simulink model "ATRIAS_vnmc"  (R2015a)
settings: Solver=ode45  StartTime=0.0  StopTime=60  FixedStep=1e-3  MinStep=1e-6  RelTol=1e-3  AbsTol=1e-4
values from neighbouring files (symbols this model uses):
  initial_boom_yaw = initial_boom_yaw + delta_yaw0    [run_model.m]
  max_floor_diff = cost_fun_opts.max_floor_diff    [opt_cmaes.m]    (also in run_model.m; set_all_params_simple.m = 0)
  noise_on_off = cost_fun_opts.noise_on_off    [opt_cmaes.m]    (also in run_model.m; set_all_params_simple.m = 0)
  noise_seed = cost_fun_opts.noise_seed    [opt_cmaes.m]    (also in run_model.m; set_all_params_simple.m = 1)
  noise_variance = cost_fun_opts.noise_variance    [opt_cmaes.m]    (also in run_model.m; set_all_params_simple.m = 0.000174532925199)
  SEA_swing_ctrl_on_off = cost_fun_opts.SEA_swing_ctrl_on_off    [opt_cmaes.m]    (also in run_model.m; set_all_params_simple.m = 0)
  sim_t = simout.twalk    [run_model.m]
  steady_dist = cost_fun_opts.steady_dist    [opt_cmaes.m]    (also in run_model.m; set_all_params_simple.m = 10)
  ts_anim = 0.0333    [run_model.m]
undefined symbols (not defined in the file or in its folder): A1_notch_f1, A2_notch_f1, A_lpf_dtau, A_lpf_velocity, B1_lpf_dtau, B1_lpf_velocity, B1_notch_f1, B2_lpf_dtau, B2_lpf_velocity, B2_notch_f1, b_hmotor, b_leg_spring, b_rotor, base_color_d, boom_color_d, boom_mount_to_center_diagonal, breakaway_friction, c, c_jointstop, com_height_offset, contactThr, coulomb_friction, CtrlPar_theta0, D12_S, D12_T, d_com, ddx_max, ddy_max, delta_phi_max, delta_phi_max_buffer, delta_phi_max_dropoff, delta_phi_min, des_forward_velocity, DS_width, dtau_des_max, dtheta0_vmc, dx0_vmc, dy_max, eref, fblink_color_d, fcut_acceleration, floor_color_d, floor_tile_width, floor_zero_height, FmaxBFSH, FmaxGLU, FmaxHAM, FmaxHFL, FmaxRF, FmaxVAS, FPCtrlPar, friction_linear_zone, g, gain_nodes_sea_torque, gamma_stance_thr, gamma_swing_thr, hip_height, HIP_MTR_MAX_CONT_TORQUE, HIP_MTR_MAX_TORQUE, hshaft_color_d ... (+236)
libraries: sm_lib x280, nesl_utility x174, simulink x114, simulink_extras x58, fl_lib x16, mblibv1 x2, dspswit3 x2
(part 2 of 23)

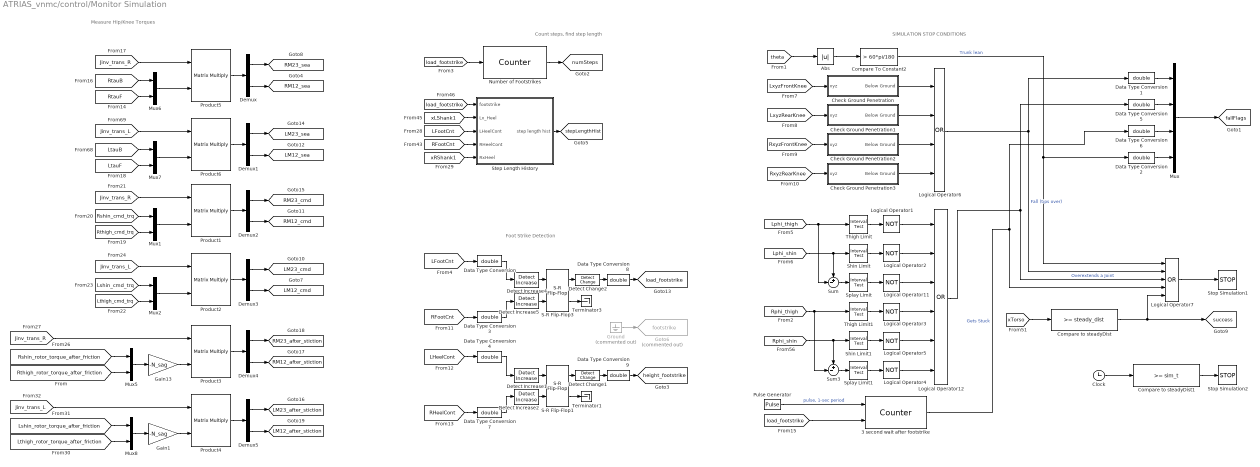
== system ATRIAS_vnmc/control/Monitor Simulation ==
  note: Foot Strike Detection
  note: Count steps, find step length
  note: SIMULATION STOP CONDITIONS
  note: Measure Hip/Knee Torques
  3 second wait after footstrike : dspswit3/Counter  Direction=Up  CountEvent=Rising edge  CounterSize=User defined  MaxCount=255  InitialCount=0  Output=Hit  HitValue=4  ResetInput=on  SamplesPerFrame=1  Ts=1  CntDtype=double  HitDtype=Boolean
  Abs : Abs
  Check Ground Penetration : Subsystem
  Check Ground Penetration1 : Subsystem
  Check Ground Penetration2 : Subsystem
  Check Ground Penetration3 : Subsystem
  Clock : Clock
  Compare To Constant2 : simulink/Logic and Bit Operations/Compare To Constant  relop=>  const=60*pi/180  OutDataTypeStr=boolean
  Compare to steadyDist : simulink/Logic and Bit Operations/Compare To Constant  relop=>=  const=steady_dist  OutDataTypeStr=boolean
  Compare to steadyDist1 : simulink/Logic and Bit Operations/Compare To Constant  relop=>=  const=sim_t  OutDataTypeStr=boolean
  Data Type Conversion{,1..9} (10 alike) : DataTypeConversion  OutDataTypeStr=double
  Demux{,1..5} (6 alike) : Demux  Outputs=2
  Detect Change1 : simulink/Logic and Bit Operations/Detect Change  vinit=0  InputProcessing=Inherited  OutDataTypeStr=boolean
  Detect Change2 : simulink/Logic and Bit Operations/Detect Change  vinit=0  InputProcessing=Inherited  OutDataTypeStr=boolean
  Detect Increase{1..2,4..5} (4 alike) : simulink/Logic and Bit Operations/Detect Increase  vinit=0.0  InputProcessing=Inherited  OutDataTypeStr=boolean
  Gain1 : Gain  Gain=-N_sag
  Gain13 : Gain  Gain=-N_sag
  Goto6 : Goto  Commented=on  GotoTag=footstrike  TagVisibility=global
  Ground : Ground  Commented=on
  Logical Operator{1..5,11} (6 alike) : Logic  Operator=NOT  AllPortsSameDT=off  OutDataTypeStr=boolean
  Logical Operator12 : Logic  Operator=OR  Inputs=6  AllPortsSameDT=off  OutDataTypeStr=boolean
  Logical Operator6 : Logic  Operator=OR  Inputs=4  AllPortsSameDT=off  OutDataTypeStr=boolean
  Logical Operator7 : Logic  Operator=OR  Inputs=5  AllPortsSameDT=off  OutDataTypeStr=boolean
  Mux : Mux
  Mux{1..2,5..8} (6 alike) : Mux  Inputs=2
  Number of Footstrikes : dspswit3/Counter  Direction=Up  CountEvent=Rising edge  CounterSize=User defined  MaxCount=255  InitialCount=0  Output=Count  HitValue=4  ResetInput=off  SamplesPerFrame=1  Ts=1  CntDtype=double  HitDtype=Boolean
  Product{1..6} (6 alike) : Product  Multiplication=Matrix(*)  InputSameDT=on
  Pulse Generator : DiscretePulseGenerator  PulseType=Time based  Period=1  PulseWidth=5
  S-R Flip-Flop1 : simulink_extras/Flip Flops/S-R Flip-Flop  initial_condition=1
  S-R Flip-Flop3 : simulink_extras/Flip Flops/S-R Flip-Flop  initial_condition=1
  Shin Limit : simulink/Logic and Bit Operations/Interval Test  IntervalClosedRight=on  uplimit=phi_shin_max  IntervalClosedLeft=on  lowlimit=phi_shin_min  OutDataTypeStr=boolean
  Shin Limit1 : simulink/Logic and Bit Operations/Interval Test  IntervalClosedRight=on  uplimit=phi_shin_max  IntervalClosedLeft=on  lowlimit=phi_shin_min  OutDataTypeStr=boolean
  Splay Limit : simulink/Logic and Bit Operations/Interval Test  IntervalClosedRight=on  uplimit=delta_phi_max  IntervalClosedLeft=on  lowlimit=delta_phi_min  OutDataTypeStr=boolean
  Splay Limit1 : simulink/Logic and Bit Operations/Interval Test  IntervalClosedRight=on  uplimit=delta_phi_max  IntervalClosedLeft=on  lowlimit=delta_phi_min  OutDataTypeStr=boolean
  Step Length History : Subsystem
  Stop Simulation1 : Stop
  Stop Simulation2 : Stop
  Sum : Sum  Inputs=+-|
  Sum3 : Sum  Inputs=+-|
  Terminator1 : Terminator
  Terminator3 : Terminator
  Thigh Limit : simulink/Logic and Bit Operations/Interval Test  IntervalClosedRight=on  uplimit=phi_thigh_max  IntervalClosedLeft=on  lowlimit=phi_thigh_min  OutDataTypeStr=boolean
  Thigh Limit1 : simulink/Logic and Bit Operations/Interval Test  IntervalClosedRight=on  uplimit=phi_thigh_max  IntervalClosedLeft=on  lowlimit=phi_thigh_min  OutDataTypeStr=boolean
  tag scope: LM12_after_stiction=global, LM12_cmd=global, LM12_sea=global, LM23_after_stiction=global, LM23_cmd=global, LM23_sea=global, RM12_after_stiction=global, RM12_cmd=global, RM12_sea=global, RM23_after_stiction=global, RM23_cmd=global, RM23_sea=global, fallFlags=global, height_footstrike=global, load_footstrike=global, numSteps=global, stepLengthHist=global, success=global
  wires:
  [theta] -> Abs/1
  Mux/1 -> [fallFlags]
  Pulse Generator/1 -> 3 second wait after footstrike/1  "pulse, 1-sec period"
  [load_footstrike] -> 3 second wait after footstrike/2
  Logical Operator6/1 -> Logical Operator7/2, Data Type Conversion1/1  "Fall (tips over)"
  Logical Operator12/1 -> Logical Operator7/3, Data Type Conversion5/1  "Overextends a Joint"
  3 second wait after footstrike/1 -> Logical Operator7/4, Data Type Conversion6/1  "Gets Stuck"
  [load_footstrike] -> Number of Footstrikes/1
  Number of Footstrikes/1 -> [numSteps]
  [load_footstrike] -> Step Length History/1(footstrike)
  [xLShank1] -> Step Length History/2(Lx_Heel)
  [LFootCnt] -> Step Length History/3(LHeelCont)
  [RFootCnt] -> Step Length History/4(RHeelCont)
  [xRShank1] -> Step Length History/5(RxHeel)
  Step Length History/1(step length hist) -> [stepLengthHist]
  [xTorso] -> Compare to steadyDist/1
  Compare to steadyDist/1 -> Logical Operator7/5, [success]
  Logical Operator7/1 -> Stop Simulation1/1
  Splay Limit/1 -> Logical Operator11/1
  Thigh Limit/1 -> Logical Operator1/1
  Shin Limit/1 -> Logical Operator2/1
  Logical Operator1/1 -> Logical Operator12/1
  Logical Operator2/1 -> Logical Operator12/2
  Logical Operator11/1 -> Logical Operator12/3
  Logical Operator3/1 -> Logical Operator12/4
  Logical Operator5/1 -> Logical Operator12/5
  Logical Operator4/1 -> Logical Operator12/6
  Splay Limit1/1 -> Logical Operator4/1
  Thigh Limit1/1 -> Logical Operator3/1
  Shin Limit1/1 -> Logical Operator5/1
  [Lphi_thigh] -> Thigh Limit/1, Sum/2
  [Lphi_shin] -> Shin Limit/1, Sum/1
  Sum/1 -> Splay Limit/1
  [Rphi_thigh] -> Sum3/2, Thigh Limit1/1
  [Rphi_shin] -> Sum3/1, Shin Limit1/1
  Sum3/1 -> Splay Limit1/1
  [LxyzFrontKnee] -> Check Ground Penetration/1(xyz)
  [RxyzRearKnee] -> Check Ground Penetration3/1(xyz)
  [RxyzFrontKnee] -> Check Ground Penetration2/1(xyz)
  [LxyzRearKnee] -> Check Ground Penetration1/1(xyz)
  Check Ground Penetration/1(Below Ground) -> Logical Operator6/1
  Check Ground Penetration1/1(Below Ground) -> Logical Operator6/2
  Check Ground Penetration2/1(Below Ground) -> Logical Operator6/3
  Check Ground Penetration3/1(Below Ground) -> Logical Operator6/4
  Compare To Constant2/1 -> Logical Operator7/1, Data Type Conversion2/1  "Trunk lean"
  Data Type Conversion1/1 -> Mux/1
  Data Type Conversion6/1 -> Mux/3
  Data Type Conversion5/1 -> Mux/2
  Data Type Conversion2/1 -> Mux/4
  Abs/1 -> Compare To Constant2/1
  [LFootCnt] -> Data Type Conversion/1
  [RFootCnt] -> Data Type Conversion3/1
  Detect Increase4/1 -> S-R Flip-Flop3/1
  Detect Increase5/1 -> S-R Flip-Flop3/2
  Detect Change2/1 -> Data Type Conversion8/1
  S-R Flip-Flop3/1 -> Detect Change2/1
  S-R Flip-Flop3/2 -> Terminator3/1
  Data Type Conversion8/1 -> [load_footstrike]
  Data Type Conversion/1 -> Detect Increase4/1
  Data Type Conversion3/1 -> Detect Increase5/1
  [LHeelCont] -> Data Type Conversion4/1
  [RHeelCont] -> Data Type Conversion7/1
  Detect Increase1/1 -> S-R Flip-Flop1/1
  Detect Increase2/1 -> S-R Flip-Flop1/2
  Detect Change1/1 -> Data Type Conversion9/1
  S-R Flip-Flop1/1 -> Detect Change1/1
  S-R Flip-Flop1/2 -> Terminator1/1
  Data Type Conversion9/1 -> [height_footstrike]
  Data Type Conversion4/1 -> Detect Increase1/1
  Data Type Conversion7/1 -> Detect Increase2/1
  Ground/1 -> Goto6/1
  [RtauB] -> Mux6/1
  [RtauF] -> Mux6/2
  Mux6/1 -> Product5/2
  [Jinv_trans_R] -> Product5/1
  Product5/1 -> Demux/1
  Demux/2 -> [RM12_sea]
  Demux/1 -> [RM23_sea]
  [LtauB] -> Mux7/1
  [LtauF] -> Mux7/2
  Mux7/1 -> Product6/2
  [Jinv_trans_L] -> Product6/1
  Product6/1 -> Demux1/1
  Demux1/2 -> [LM12_sea]
  Demux1/1 -> [LM23_sea]
  [Rshin_cmd_trq] -> Mux1/1
  [Rthigh_cmd_trq] -> Mux1/2
  Mux1/1 -> Product1/2
  [Jinv_trans_R] -> Product1/1
  Product1/1 -> Demux2/1
  Demux2/2 -> [RM12_cmd]
  Demux2/1 -> [RM23_cmd]
  [Lshin_cmd_trq] -> Mux2/1
  [Lthigh_cmd_trq] -> Mux2/2
  Mux2/1 -> Product2/2
  [Jinv_trans_L] -> Product2/1
  Product2/1 -> Demux3/1
  Demux3/2 -> [LM12_cmd]
  Demux3/1 -> [LM23_cmd]
  Clock/1 -> Compare to steadyDist1/1
  Compare to steadyDist1/1 -> Stop Simulation2/1
  [Jinv_trans_R] -> Product3/1
  Product3/1 -> Demux4/1
  Demux4/2 -> [RM12_after_stiction]
  Demux4/1 -> [RM23_after_stiction]
  [Jinv_trans_L] -> Product4/1
  Product4/1 -> Demux5/1
  Demux5/2 -> [LM12_after_stiction]
  Demux5/1 -> [LM23_after_stiction]
  [Rshin_rotor_torque_after_friction] -> Mux5/1
  [Rthigh_rotor_torque_after_friction] -> Mux5/2
  Mux5/1 -> Gain13/1
  [Lshin_rotor_torque_after_friction] -> Mux8/1
  [Lthigh_rotor_torque_after_friction] -> Mux8/2
  Mux8/1 -> Gain1/1
  Gain13/1 -> Product3/2
  Gain1/1 -> Product4/2

== system ATRIAS_vnmc/control/Plot Signals ==
  note: Virtual Torques
  note: GRFs, Leg Load,
      | Contact
  note: Virtual Joint Angles
  note: Robot Joint Angles
  note: Joint Torques
  note: Global Marker Positions
  note: Muscle States
  note: Individual Muscles
  note: Stimulations
  note: Muscle Lce,
      | Moment Arms
  note: Compare Continuous
      | to Discrete Angles
  note: VMC
  Discrete-Continuous Plots : Subsystem
  "GRFs, leg load, contact" : Subsystem
  Markers : Subsystem
  Robot Angles : Subsystem
  Torques : Subsystem
  VMC Plots : Subsystem
  Virtual Angles : Subsystem
  individual muscles : Subsystem
  muscle comparison : Subsystem
  muscle etc : Subsystem
  stims : Subsystem  Commented=on
  virtual joint torques : Subsystem

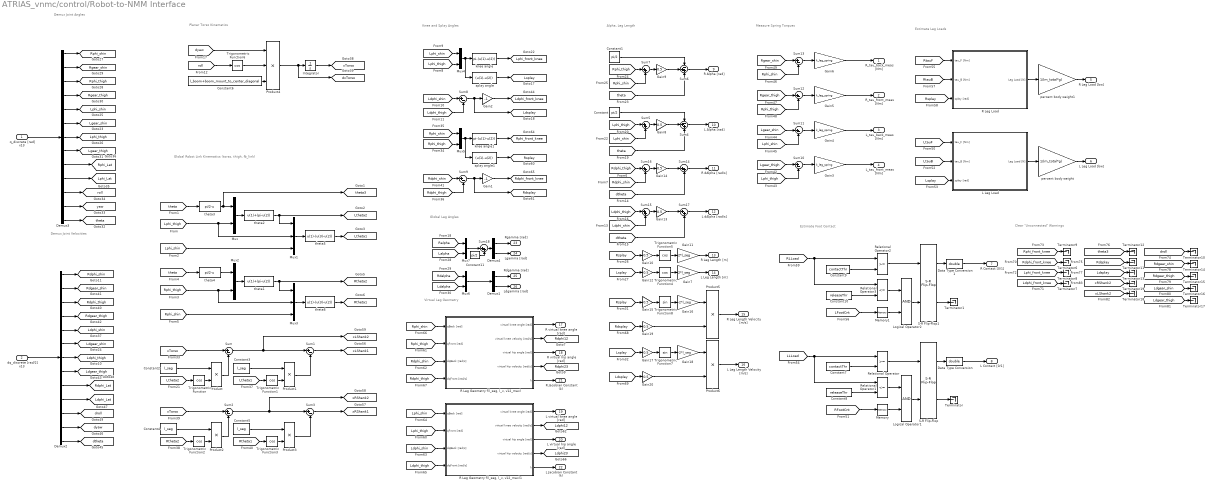
== system ATRIAS_vnmc/control/Robot-to-NMM Interface ==
  note: Global Robot Link Kinematics
      | (torso, thigh, fb_link)
  note: Planar Torso Kinematics
  note: Alpha, Leg Length
  note: Demux Joint
      | Angles
  note: Demux Joint
      | Velocities
  note: Knee and Splay Angles
  note: Virtual Leg Geometry
  note: Measure Spring Torques
  note: Estimate Leg Loads
  note: Estimate Foot Contact
  note: Clear "Unconnected" Warnings
  note: Global Leg Angles
  q_discrete [rad] x13 : Inport
  dq_discrete [rad/2] x13 : Inport  Port=2
  Constant : Constant  Value=pi/2
  Constant1 : Constant  Value=pi/2
  Constant10 : Constant  Value=releaseThr
  Constant11 : Constant  Value=pi/2
  Constant{2..5} (4 alike) : Constant  Value=l_seg
  Constant6 : Constant  Value=l_boom+boom_mount_to_center_diagonal
  Constant7 : Constant  Value=contactThr
  Constant8 : Constant  Value=releaseThr
  Constant9 : Constant  Value=contactThr
  Data Type Conversion : DataTypeConversion  OutDataTypeStr=double
  Data Type Conversion1 : DataTypeConversion  OutDataTypeStr=double
  Demux1 : Demux  Outputs=2
  Demux2 : Demux  Outputs=13
  Demux3 : Demux  Outputs=13
  Demux4 : Demux  Outputs=2
  Gain1 : Gain  Gain=-1
  Gain{8..10,12..15,17,19..20} (10 alike) : Gain  Gain=0.5
  Gain11 : Gain  Gain=2*l_seg
  Gain16 : Gain  Gain=-2*l_seg
  Gain18 : Gain  Gain=-2*l_seg
  Gain2 : Gain  Gain=-1
  Gain{3..6} (4 alike) : Gain  Gain=k_leg_spring
  Gain7 : Gain  Gain=2*l_seg
  Integrator : Integrator
  L Leg Load : Subsystem
  Logical Operator1 : Logic  AllPortsSameDT=off  OutDataTypeStr=boolean
  Logical Operator2 : Logic  AllPortsSameDT=off  OutDataTypeStr=boolean
  Memory : Memory
  Memory1 : Memory
  Mux{,2,4..7} (6 alike) : Mux  Inputs=2
  Mux1 : Mux  Inputs=3
  Mux3 : Mux  Inputs=3
  Product{,1..3,5..6} (6 alike) : Product
  Product4 : Product  Inputs=3
  "R Leg Geometry f(l_seg, l_v, v12_max)" : Subsystem
  "R Leg Geometry f(l_seg, l_v, v12_max)1" : Subsystem
  R Leg Load : Subsystem
  Relational Operator : RelationalOperator  OutDataTypeStr=boolean
  Relational Operator1 : RelationalOperator  Operator=<=  OutDataTypeStr=boolean
  Relational Operator2 : RelationalOperator  OutDataTypeStr=boolean
  Relational Operator3 : RelationalOperator  Operator=<=  OutDataTypeStr=boolean
  S-R Flip-Flop : simulink_extras/Flip Flops/S-R Flip-Flop  initial_condition=0
  S-R Flip-Flop1 : simulink_extras/Flip Flops/S-R Flip-Flop  initial_condition=0
  Sum{,1..3,8..13} (10 alike) : Sum  Inputs=|+-
  Sum{5,7,14..18} (7 alike) : Sum  Inputs=|++
  Sum4 : Sum  Inputs=-++
  Sum6 : Sum  Inputs=-++
  Terminator{,1,6..19} (16 alike) : Terminator
  Trigonometric Function{,1..6} (7 alike) : Trigonometry  Operator=cos
  Trigonometric Function7 : Trigonometry
  Trigonometric Function8 : Trigonometry
  knee angle : Fcn  Expr=pi-(u(1)-u(2))
  knee angle1 : Fcn  Expr=pi-(u(1)-u(2))
  percent body weight : Gain  Gain=1/(m_total*g)
  percent body weight1 : Gain  Gain=1/(m_total*g)
  splay angle : Fcn  Expr=(u(1)-u(2))
  splay angle1 : Fcn  Expr=(u(1)-u(2))
  theta1 : Fcn  Expr=u(1)+(pi-u(2))
  theta2 : Fcn  Expr=u(1)+(pi-u(2))
  theta3 : Fcn  Expr=pi/2-u
  theta4 : Fcn  Expr=pi/2-u
  theta5 : Fcn  Expr=u(1)-(u(3)-u(2))
  theta6 : Fcn  Expr=u(1)-(u(3)-u(2))
  R_tau_back_meas [Nm] : Outport
  R_tau_front_meas [Nm] : Outport  Port=2
  L_tau_back_meas [Nm] : Outport  Port=3
  L_tau_front_meas [Nm] : Outport  Port=4
  R Leg Load [bw] : Outport  Port=5
  L Leg Load [bw] : Outport  Port=6
  R Contact [0/1] : Outport  Port=7
  L Contact [0/1] : Outport  Port=8
  R Alpha [rad] : Outport  Port=9
  L Alpha [rad] : Outport  Port=10
  R dAlpha [rad/s] : Outport  Port=11
  L dAlpha [rad/s] : Outport  Port=12
  R Leg Length [m] : Outport  Port=13
  L Leg Length [m] : Outport  Port=14
  R Leg Length Velocity [m/s] : Outport  Port=15
  L Leg Length Velocity [m/s] : Outport  Port=16
  R virtual knee angle [rad] : Outport  Port=17
  R virtual hip angle [rad] : Outport  Port=18
  L virtual knee angle [rad] : Outport  Port=19
  L virtual hip angle [rad] : Outport  Port=20
  R Jacobian Constant (k) : Outport  Port=21
  L Jacobian Constant (k) : Outport  Port=22
  Rgamma [rad] : Outport  Port=23
  Lgamma [rad] : Outport  Port=24
  Rdgamma [rad] : Outport  Port=25
  Ldgamma [rad] : Outport  Port=26
  tag scope: Ldgear_shin=global, Ldgear_thigh=global, Ldphi12=global, Ldphi23=global, Ldphi_Lat=global, Ldphi_front_knee=global, Ldphi_shin=global, Ldphi_thigh=global, Ldsplay=global, Lgear_shin=global, Lgear_thigh=global, Lphi_Lat=global, Lphi_front_knee=global, Lphi_shin=global, Lphi_thigh=global, Lsplay=global, Ltheta1=global, Ltheta2=global, Rdgear_shin=global, Rdgear_thigh=global, Rdphi12=global, Rdphi23=global, Rdphi_Lat=global, Rdphi_front_knee=global, Rdphi_shin=global, Rdphi_thigh=global, Rdsplay=global, Rgear_shin=global, Rgear_thigh=global, Rphi_Lat=global, Rphi_front_knee=global, Rphi_shin=global, Rphi_thigh=global, Rsplay=global, Rtheta1=global, Rtheta2=global, droll=global, dtheta=global, dxTorso=global, dyaw=global, roll=global, theta3=global, theta=global, xLShank1=global, xLShank2=global, xRShank1=global, xRShank2=global, xTorso=global, yaw=global
  wires:
  Sum3/1 -> [xRShank1]
  Sum2/1 -> [xRShank2], Sum3/1
  Product3/1 -> Sum3/2
  Trigonometric Function3/1 -> Product3/2
  Constant2/1 -> Product/1
  Trigonometric Function/1 -> Product/2
  Sum1/1 -> [xLShank1]
  Constant3/1 -> Product1/1
  Trigonometric Function2/1 -> Product2/2
  Product1/1 -> Sum1/2
  [Rtheta2] -> Trigonometric Function2/1
  Sum/1 -> [xLShank2], Sum1/1
  [Ltheta1] -> Trigonometric Function1/1
  Product/1 -> Sum/2
  Product2/1 -> Sum2/2
  [xTorso] -> Sum2/1
  [Rtheta1] -> Trigonometric Function3/1
  Constant4/1 -> Product2/1
  Constant5/1 -> Product3/1
  [xTorso] -> Sum/1
  [Ltheta2] -> Trigonometric Function/1
  Product4/1 -> [dxTorso], Integrator/1
  Trigonometric Function1/1 -> Product1/2
  Integrator/1 -> [xTorso]
  [dyaw] -> Product4/1
  [theta] -> theta3/1
  [Lphi_thigh] -> Mux1/2, Mux/2
  theta3/1 -> Mux/1, [theta3]
  Mux/1 -> theta2/1
  theta2/1 -> Mux1/1, [Ltheta2]
  Mux1/1 -> theta5/1
  [Lphi_shin] -> Mux1/3
  [theta] -> theta4/1
  [Rphi_thigh] -> Mux3/2, Mux2/2
  theta4/1 -> Mux2/1
  Mux2/1 -> theta1/1
  theta1/1 -> Mux3/1, [Rtheta2]
  Mux3/1 -> theta6/1
  [Rphi_shin] -> Mux3/3
  theta5/1 -> [Ltheta1]
  theta6/1 -> [Rtheta1]
  [theta] -> Sum4/3
  Constant/1 -> Sum4/1
  [Lphi_thigh] -> Sum5/1
  [Lphi_shin] -> Sum5/2
  Sum5/1 -> Gain8/1
  Gain8/1 -> Sum4/2
  Sum4/1 -> L Alpha [rad]/1
  [theta] -> Sum6/3
  Constant1/1 -> Sum6/1
  [Rphi_thigh] -> Sum7/1
  [Rphi_shin] -> Sum7/2
  Sum7/1 -> Gain9/1
  Gain9/1 -> Sum6/2
  Sum6/1 -> R Alpha [rad]/1
  Gain12/1 -> Trigonometric Function4/1
  Gain10/1 -> Trigonometric Function5/1
  Trigonometric Function4/1 -> Gain7/1
  Trigonometric Function5/1 -> Gain11/1
  Demux3/1 -> [Rphi_shin]
  Demux3/2 -> [Rgear_shin]
  Demux3/3 -> [Rphi_thigh]
  Demux3/4 -> [Rgear_thigh]
  Demux3/5 -> [Lphi_shin]
  Demux3/6 -> [Lgear_shin]
  Demux3/7 -> [Lphi_thigh]
  Demux3/8 -> [Lgear_thigh]
  Demux3/9 -> [Rphi_Lat]
  Demux3/10 -> [Lphi_Lat]
  Demux3/11 -> [roll]
  Demux3/12 -> [yaw]
  Demux3/13 -> [theta]
  Demux2/13 -> [dtheta]
  Demux2/8 -> [Ldgear_thigh]
  Demux2/10 -> [Ldphi_Lat]
  Demux2/6 -> [Ldgear_shin]
  Demux2/9 -> [Rdphi_Lat]
  Demux2/11 -> [droll]
  Demux2/12 -> [dyaw]
  Demux2/4 -> [Rdgear_thigh]
  Demux2/5 -> [Ldphi_shin]
  Demux2/7 -> [Ldphi_thigh]
  Demux2/1 -> [Rdphi_shin]
  Demux2/3 -> [Rdphi_thigh]
  Demux2/2 -> [Rdgear_shin]
  q_discrete [rad] x13/1 -> Demux3/1
  dq_discrete [rad/2] x13/1 -> Demux2/1
  Mux4/1 -> splay angle/1, knee angle/1
  [Lphi_thigh] -> Mux4/2
  [Lphi_shin] -> Mux4/1
  knee angle/1 -> [Lphi_front_knee]
  [Ldphi_thigh] -> Sum8/2
  [Ldphi_shin] -> Sum8/1
  Sum8/1 -> [Ldsplay], Gain2/1
  Gain2/1 -> [Ldphi_front_knee]
  splay angle/1 -> [Lsplay]
  Trigonometric Function6/1 -> Product4/2
  [roll] -> Trigonometric Function6/1
  Constant6/1 -> Product4/3
  Mux5/1 -> splay angle1/1, knee angle1/1
  [Rphi_thigh] -> Mux5/2
  [Rphi_shin] -> Mux5/1
  knee angle1/1 -> [Rphi_front_knee]
  [Rdphi_thigh] -> Sum9/2
  [Rdphi_shin] -> Sum9/1
  Sum9/1 -> [Rdsplay], Gain1/1
  Gain1/1 -> [Rdphi_front_knee]
  splay angle1/1 -> [Rsplay]
  [Lgear_shin] -> Sum11/1
  Sum11/1 -> Gain4/1
  [Lphi_shin] -> Sum11/2
  Gain4/1 -> L_tau_back_meas [Nm]/1
  [Lgear_thigh] -> Sum10/1
  Sum10/1 -> Gain3/1
  [Lphi_thigh] -> Sum10/2
  Gain3/1 -> L_tau_front_meas [Nm]/1
  [Rgear_shin] -> Sum13/1
  Sum13/1 -> Gain6/1
  [Rphi_shin] -> Sum13/2
  Gain6/1 -> R_tau_back_meas [Nm]/1
  [Rgear_thigh] -> Sum12/1
  Sum12/1 -> Gain5/1
  [Rphi_thigh] -> Sum12/2
  Gain5/1 -> R_tau_front_meas [Nm]/1
  [Lsplay] -> L Leg Load/3(splay [rad])
  L Leg Load/1(Leg Load [N]) -> percent body weight/1
  [LtauF] -> L Leg Load/1(tau_F [Nm])
  [LtauB] -> L Leg Load/2(tau_B [Nm])
  percent body weight/1 -> L Leg Load [bw]/1
  Relational Operator/1 -> S-R Flip-Flop/1
  Constant7/1 -> Relational Operator/2
  S-R Flip-Flop/2 -> Terminator/1
  Logical Operator1/1 -> S-R Flip-Flop/2
  [RFootCnt] -> Memory/1
  Constant8/1 -> Relational Operator1/2
  Relational Operator1/1 -> Logical Operator1/1
  Memory/1 -> Logical Operator1/2
  Data Type Conversion/1 -> L Contact [0/1]/1
  S-R Flip-Flop/1 -> Data Type Conversion/1
  [LLLoad] -> Relational Operator/1, Relational Operator1/1
  [Rsplay] -> R Leg Load/3(splay [rad])
  R Leg Load/1(Leg Load [N]) -> percent body weight1/1
  [RtauF] -> R Leg Load/1(tau_F [Nm])
  [RtauB] -> R Leg Load/2(tau_B [Nm])
  percent body weight1/1 -> R Leg Load [bw]/1
  Relational Operator2/1 -> S-R Flip-Flop1/1
  Constant9/1 -> Relational Operator2/2
  S-R Flip-Flop1/2 -> Terminator1/1
  Logical Operator2/1 -> S-R Flip-Flop1/2
  [LFootCnt] -> Memory1/1
  Constant10/1 -> Relational Operator3/2
  Relational Operator3/1 -> Logical Operator2/1
  Memory1/1 -> Logical Operator2/2
  Data Type Conversion1/1 -> R Contact [0/1]/1
  S-R Flip-Flop1/1 -> Data Type Conversion1/1
  [RLLoad] -> Relational Operator3/1, Relational Operator2/1
  [Rsplay] -> Gain10/1
  [Lsplay] -> Gain12/1
  Gain11/1 -> R Leg Length [m]/1
  Gain7/1 -> L Leg Length [m]/1
  [Rphi_thigh] -> "R Leg Geometry f(l_seg, l_v, v12_max)"/2(qFront [rad])
  [Rphi_shin] -> "R Leg Geometry f(l_seg, l_v, v12_max)"/1(qBack [rad])
  [Rdphi_shin] -> "R Leg Geometry f(l_seg, l_v, v12_max)"/3(dqBack [rad/s])
  [Rdphi_thigh] -> "R Leg Geometry f(l_seg, l_v, v12_max)"/4(dqFront [rad/s])
  "R Leg Geometry f(l_seg, l_v, v12_max)"/4(virtual hip velocity [rad/s]) -> [Rdphi23]
  "R Leg Geometry f(l_seg, l_v, v12_max)"/2(virtual knee velocity [rad/s]) -> [Rdphi12]
  "R Leg Geometry f(l_seg, l_v, v12_max)"/5(k) -> R Jacobian Constant (k)/1
  [Lphi_thigh] -> "R Leg Geometry f(l_seg, l_v, v12_max)1"/2(qFront [rad])
  [Lphi_shin] -> "R Leg Geometry f(l_seg, l_v, v12_max)1"/1(qBack [rad])
  [Ldphi_shin] -> "R Leg Geometry f(l_seg, l_v, v12_max)1"/3(dqBack [rad/s])
  [Ldphi_thigh] -> "R Leg Geometry f(l_seg, l_v, v12_max)1"/4(dqFront [rad/s])
  "R Leg Geometry f(l_seg, l_v, v12_max)1"/5(k) -> L Jacobian Constant (k)/1
  "R Leg Geometry f(l_seg, l_v, v12_max)"/3(virtual hip angle [rad]) -> R virtual hip angle [rad]/1
  "R Leg Geometry f(l_seg, l_v, v12_max)"/1(virtual knee angle [rad]) -> R virtual knee angle [rad]/1
  "R Leg Geometry f(l_seg, l_v, v12_max)1"/1(virtual knee angle [rad]) -> L virtual knee angle [rad]/1
  "R Leg Geometry f(l_seg, l_v, v12_max)1"/3(virtual hip angle [rad]) -> L virtual hip angle [rad]/1
  "R Leg Geometry f(l_seg, l_v, v12_max)1"/2(virtual knee velocity [rad/s]) -> [Ldphi12]
  "R Leg Geometry f(l_seg, l_v, v12_max)1"/4(virtual hip velocity [rad/s]) -> [Ldphi23]
  [Rdphi_front_knee] -> Terminator6/1
  [Ldphi_front_knee] -> Terminator7/1
  [Lphi_front_knee] -> Terminator8/1
  [Rphi_front_knee] -> Terminator9/1
  [droll] -> Terminator10/1
  [Rdsplay] -> Terminator11/1
  [theta3] -> Terminator12/1
  [Ldsplay] -> Terminator13/1
  [Rdgear_shin] -> Terminator14/1
  [Rdgear_thigh] -> Terminator15/1
  [Ldgear_shin] -> Terminator16/1
  [Ldgear_thigh] -> Terminator17/1
  [xLShank2] -> Terminator18/1
  [xRShank2] -> Terminator19/1
  Sum17/1 -> L dAlpha [rad/s]/1
  Sum14/1 -> R dAlpha [rad/s]/1
  [Ldphi_thigh] -> Sum15/1
  [Ldphi_shin] -> Sum15/2
  Sum15/1 -> Gain13/1
  Gain13/1 -> Sum17/1
  [dtheta] -> Sum17/2
  [Rdphi_thigh] -> Sum16/1
  [Rdphi_shin] -> Sum16/2
  Sum16/1 -> Gain14/1
  Gain14/1 -> Sum14/1
  [dtheta] -> Sum14/2
  Constant11/1 -> Sum18/2
  [Ralpha] -> Mux7/1
  [Lalpha] -> Mux7/2
  Mux7/1 -> Sum18/1
  Sum18/1 -> Demux4/1
  Demux4/1 -> Rgamma [rad]/1
  Demux4/2 -> Lgamma [rad]/1
  [Rdalpha] -> Mux6/1
  [Ldalpha] -> Mux6/2
  Mux6/1 -> Demux1/1
  Demux1/1 -> Rdgamma [rad]/1
  Demux1/2 -> Ldgamma [rad]/1
  Gain15/1 -> Trigonometric Function8/1
  Trigonometric Function8/1 -> Gain16/1
  [Rsplay] -> Gain15/1
  Gain16/1 -> Product5/1
  [Rdsplay] -> Gain19/1
  Gain19/1 -> Product5/2
  Product5/1 -> R Leg Length Velocity [m/s]/1
  Gain17/1 -> Trigonometric Function7/1
  Trigonometric Function7/1 -> Gain18/1
  [Lsplay] -> Gain17/1
  Gain18/1 -> Product6/1
  [Ldsplay] -> Gain20/1
  Gain20/1 -> Product6/2
  Product6/1 -> L Leg Length Velocity [m/s]/1

== system ATRIAS_vnmc/control/SEA Ctrl ==
  note: Order:
      | backR
      | frontR
      | backL
      | frontL
  note: Motor Order:
      |
      | backR
      | frontR
      | latR
      | backL
      | frontL
      | latL
  Desired Torque [Nm] x6 : Inport  OutDataTypeStr=double  PortDimensions=6  SampleTime=sample_time
  Desired SEA Torque Velocity [Nm] x4 : Inport  Port=2  OutDataTypeStr=double  PortDimensions=4  SampleTime=sample_time
  Enable SEA Control [1/0] x4 : Inport  Port=3  OutDataTypeStr=boolean  PortDimensions=4  SampleTime=sample_time
  q : Inport  Port=4  OutDataTypeStr=double  PortDimensions=13  SampleTime=sample_time
  dq : Inport  Port=5  OutDataTypeStr=double  PortDimensions=13  SampleTime=sample_time
  Activate SEA Control : Subsystem
  Antiresonance Compensation : Subsystem
  Mux{1..2,4..5} (4 alike) : Mux
  Mux3 : Mux  Inputs=2
  SEA Controller (Torque) : Subsystem
  Selector1 : Selector  InputPortWidth=13  Indices=[10]
  Selector11 : Selector  InputPortWidth=13  Indices=[10]
  Selector12 : Selector  InputPortWidth=13  Indices=[5 6]
  Selector13 : Selector  InputPortWidth=13  Indices=[7 8]
  Selector14 : Selector  InputPortWidth=13  Indices=[9]
  Selector15 : Selector  InputPortWidth=13  Indices=[1 2]
  Selector16 : Selector  InputPortWidth=13  Indices=[3 4]
  Selector{17..20,25..28} (8 alike) : Selector  InputPortWidth=2  Indices=[1]
  Selector2 : Selector  InputPortWidth=13  Indices=[5 6]
  Selector{21..24,29..32} (8 alike) : Selector  InputPortWidth=2  Indices=[2]
  Selector3 : Selector  InputPortWidth=6  Indices=[3 6]
  Selector33 : Selector  InputPortWidth=6  Indices=[1 2 4 5]
  Selector4 : Selector  InputPortWidth=13  Indices=[7 8]
  Selector5 : Selector  InputPortWidth=13  Indices=[9]
  Selector6 : Selector  InputPortWidth=13  Indices=[1 2]
  Selector7 : Selector  InputPortWidth=13  Indices=[3 4]
  Selector8 : Selector  InputPortWidth=6  Indices=[1 2 5 3 4 6]
  Selector9 : Selector  InputPortWidth=6  Indices=[1 2 4 5]
  Terminator{,1..5} (6 alike) : Terminator
  Torque Limiter (outside) 1 : Saturate  UpperLimit=max_sagittal_unloaded_torque  LowerLimit=-max_sagittal_unloaded_torque
      settings: AttributesFormatString=Hi: %<UpperLimit>\nLo: %<LowerLimit>
  tau_desired_signals : Gain  Description=xPCTag(1)=tau_cmd_signal;
  tau_cmd [Nm] x6 : Outport  OutDataTypeStr=double  PortDimensions=6  SampleTime=0  InitialOutput=[0 0 0 0 0 0]
  wires:
  SEA Controller (Torque)/1(tau_cmd sagittal [Nm] x4) -> Activate SEA Control/1(SEA Control Signal [Nm] x4)
  Torque Limiter (outside) 1/1 -> Activate SEA Control/3(Torque Signal [Nm] x4)
  Desired Torque [Nm] x6/1 -> Selector33/1, Selector9/1, Selector3/1, tau_desired_signals/1
  Selector8/1 -> tau_cmd [Nm] x6/1
  tau_desired_signals/1 -> Terminator1/1
  Selector5/1 -> [qLatR]
  Selector1/1 -> [qLatL]
  Selector6/1 -> [qBackR]
  Selector7/1 -> [qFrontR]
  Selector2/1 -> [qBackL]
  Selector4/1 -> [qFrontL]
  q/1 -> Selector2/1, Selector7/1, Selector6/1, Selector4/1, Selector5/1, Selector1/1
  dq/1 -> Selector11/1, Selector14/1, Selector13/1, Selector15/1, Selector16/1, Selector12/1
  Selector14/1 -> [dqLatR]
  Selector11/1 -> [dqLatL]
  Selector15/1 -> [dqBackR]
  Selector16/1 -> [dqFrontR]
  Selector12/1 -> [dqBackL]
  Selector13/1 -> [dqFrontL]
  Mux1/1 -> SEA Controller (Torque)/1(phi_load [rad] x4)
  [qBackR] -> Selector17/1
  Selector17/1 -> Mux1/1
  Selector19/1 -> Mux1/3
  Selector18/1 -> Mux1/2
  Selector20/1 -> Mux1/4
  [qFrontR] -> Selector18/1
  [qBackL] -> Selector19/1
  [qFrontL] -> Selector20/1
  Mux2/1 -> SEA Controller (Torque)/2(phi_gear [rad] x4)
  [qBackR] -> Selector21/1
  Selector21/1 -> Mux2/1
  Selector23/1 -> Mux2/3
  Selector22/1 -> Mux2/2
  Selector24/1 -> Mux2/4
  [qFrontR] -> Selector22/1
  [qBackL] -> Selector23/1
  [qFrontL] -> Selector24/1
  Mux4/1 -> SEA Controller (Torque)/5(dphi_load [rad/s] x4)
  [dqBackR] -> Selector25/1
  Selector25/1 -> Mux4/1
  Selector27/1 -> Mux4/3
  Selector26/1 -> Mux4/2
  Selector28/1 -> Mux4/4
  [dqFrontR] -> Selector26/1
  [dqBackL] -> Selector27/1
  [dqFrontL] -> Selector28/1
  Mux5/1 -> SEA Controller (Torque)/6(dphi_gear [rad/s] x4)
  [dqBackR] -> Selector29/1
  Selector29/1 -> Mux5/1
  Selector31/1 -> Mux5/3
  Selector30/1 -> Mux5/2
  Selector32/1 -> Mux5/4
  [dqFrontR] -> Selector30/1
  [dqBackL] -> Selector31/1
  [dqFrontL] -> Selector32/1
  Selector33/1 -> SEA Controller (Torque)/3(tau_des sagittal [Nm] x4)
  Selector3/1 -> Mux3/2
  Mux3/1 -> Selector8/1
  Enable SEA Control [1/0] x4/1 -> Activate SEA Control/2("SEA on/off [1/0] x4 ")
  Selector9/1 -> Antiresonance Compensation/1(Torque)
  Desired SEA Torque Velocity [Nm] x4/1 -> SEA Controller (Torque)/4(dtau_des sagittal [Nm] x4)
  Activate SEA Control/1(Torque Command [Nm] x4) -> Mux3/1
  [dqLatL] -> Terminator/1
  [dqLatR] -> Terminator2/1
  [qLatL] -> Terminator3/1
  [qLatR] -> Terminator4/1
  Antiresonance Compensation/1(Filtered Torque) -> Torque Limiter (outside) 1/1
  SEA Controller (Torque)/2(tau_measured [Nm] x4) -> Terminator5/1

== system ATRIAS_vnmc/control/Turn on NMM ==
  Constant : Constant  Value=0
  Data Type Conversion1 : DataTypeConversion  OutDataTypeStr=boolean
  Detect Increase : simulink/Logic and Bit Operations/Detect Increase  vinit=1  InputProcessing=Inherited  OutDataTypeStr=boolean
  S-R Flip-Flop : simulink_extras/Flip Flops/S-R Flip-Flop  initial_condition=0
  Terminator : Terminator
  Turn on NMM : Outport
  tag scope: NMM_turned_on=global
  wires:
  Constant/1 -> Data Type Conversion1/1
  S-R Flip-Flop/1 -> Turn on NMM/1, [NMM_turned_on]
  [Rstance_VMC] -> Detect Increase/1
  S-R Flip-Flop/2 -> Terminator/1
  Detect Increase/1 -> S-R Flip-Flop/1
  Data Type Conversion1/1 -> S-R Flip-Flop/2

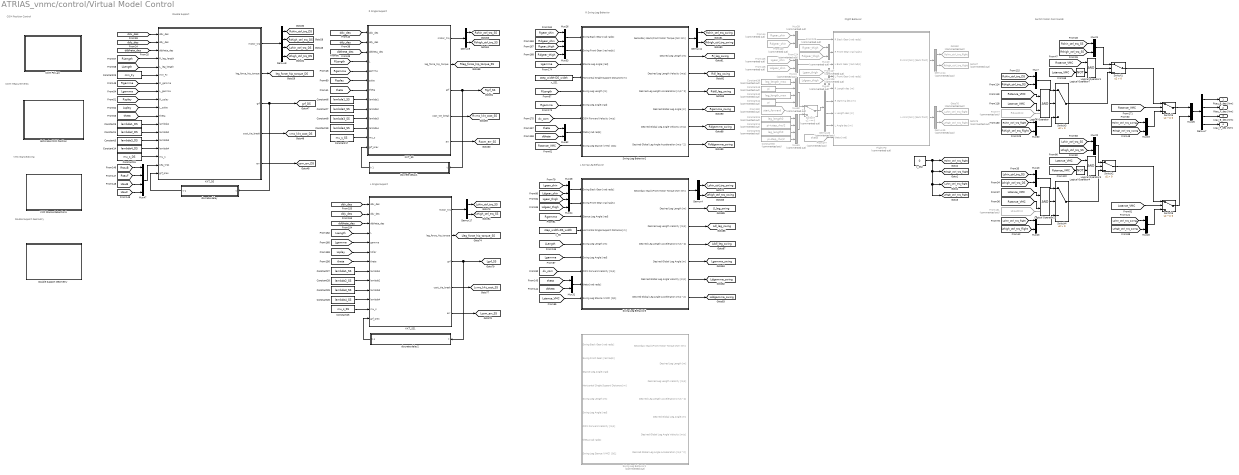
== system ATRIAS_vnmc/control/Virtual Model Control ==
  note: COM Position Control
  note: COM Measurements
  note: Double Support
  note: L Swing Leg Behavior
  note: R Single Support
  note: VMC Stance/Swing
  note: Flight Behavior
  note: L Single Support
  note: R Swing Leg Behavior
  note: Switch Motor Commands
  note: Double Support
      | Geometry
  COM PD Law : Subsystem
  Constant11 : Constant  Commented=on  Value=pi+step_rho/2
  Constant14 : Constant  Value=lambda4_DS
  Constant15 : Constant  Value=mu_s_DS
  Constant17 : Constant  Value=mu_s_SS
  Constant19 : Constant  Value=lambda4_SS
  Constant23 : Constant  Value=min_Fy
  Constant24 : Constant  Commented=on  Value=leg_length0
  Constant25 : Constant  Value=mu_s_SS
  Constant26 : Constant  Value=lambda4_SS
  Constant27 : Constant  Value=lambda1_SS
  Constant28 : Constant  Value=lambda2_SS
  Constant29 : Constant  Value=lambda3_SS
  Constant3 : Constant  Value=lambda1_DS
  Constant30 : Constant  Commented=on  Value=pi-step_rho/2
  Constant31 : Constant  Commented=on  Value=leg_length0
  Constant39 : Constant  Commented=on  Value=leg_length_max
  Constant4 : Constant  Value=lambda2_DS
  Constant40 : Constant  Commented=on  Value=leg_length_max
  Constant43 : Constant  Commented=on  Value=pi
  Constant44 : Constant  Commented=on  Value=pi
  Constant5 : Constant  Value=lambda3_DS
  Constant6 : Constant  Value=lambda1_SS
  Constant7 : Constant  Value=lambda2_SS
  Constant8 : Constant  Value=lambda3_SS
  Demux{4,9,11,17} (4 alike) : Demux  Outputs=2
  Demux14 : Demux  Commented=on  Outputs=2
  Demux15 : Demux  Commented=on  Outputs=2
  Demux20 : Demux  Commented=on
  Demux7 : Demux
  Demux8 : Demux
  Double Support Geometry : Subsystem
  Estimate COM Position : Subsystem
  Flight PD : Subsystem  Commented=on
  From120 : From  Commented=on  GotoTag=Rdgear_shin  TagVisibility=global
  From123 : From  Commented=on  GotoTag=Rgear_thigh  TagVisibility=global
  From124 : From  Commented=on  GotoTag=Rdgear_thigh  TagVisibility=global
  From125 : From  Commented=on  GotoTag=Lgear_shin  TagVisibility=global
  From126 : From  Commented=on  GotoTag=Ldgear_shin  TagVisibility=global
  From127 : From  Commented=on  GotoTag=Lgear_thigh  TagVisibility=global
  From128 : From  Commented=on  GotoTag=Ldgear_thigh  TagVisibility=global
  From131 : From  Commented=on  GotoTag=LFootCnt  TagVisibility=global
  From132 : From  Commented=on  GotoTag=start_forward  TagVisibility=global
  From177 : From  Commented=on  GotoTag=theta  TagVisibility=global
  From44 : From  Commented=on  GotoTag=Rgear_shin  TagVisibility=global
  From77 : From  Commented=on  GotoTag=RFootCnt  TagVisibility=global
  Goto27 : Goto  Commented=on  GotoTag=Rthigh_ctrl_trq_flight  TagVisibility=global
  Goto62 : Goto  Commented=on  GotoTag=Rshin_ctrl_trq_flight  TagVisibility=global
  Goto75 : Goto  Commented=on  GotoTag=Lthigh_ctrl_trq_flight  TagVisibility=global
  Goto76 : Goto  Commented=on  GotoTag=Lshin_ctrl_trq_flight  TagVisibility=global
  KKT_DS : MATLAB Function  TreatAsAtomicUnit=on
  KKT_SS : MATLAB Function  TreatAsAtomicUnit=on
  KKT_SS1 : MATLAB Function  TreatAsAtomicUnit=on
  Logical Operator{,1..3} (4 alike) : Logic  AllPortsSameDT=off  OutDataTypeStr=boolean
  Logical Operator4 : Logic  Operator=NOT  AllPortsSameDT=off  OutDataTypeStr=boolean
  Logical Operator7 : Logic  Operator=NOT  AllPortsSameDT=off  OutDataTypeStr=boolean
  Mux{7,19..26,28,31,43,52..53,60} (15 alike) : Mux  Inputs=2
  Mux{39..42} (4 alike) : Mux  Commented=on  Inputs=2
  Mux47 : Mux
  Mux61 : Mux  Commented=on
  Mux62 : Mux  Commented=on
  Swing Leg Behavior1 : Subsystem  Commented=on
  Swing Leg Behavior2 : Subsystem
  Swing Leg Behavior3 : Subsystem
  Switch{1..4} (4 alike) : Switch  Criteria=u2 > Threshold
  Switch5 : Switch  Criteria=u2 ~= 0
  Switch6 : Switch  Criteria=u2 ~= 0
  Switch7 : Switch  Commented=on  Criteria=u2 ~= 0
  VMC Stance Detection1 : Subsystem
  discrete delay : Subsystem  TreatAsAtomicUnit=on
      settings: MinAlgLoopOccurrences=on
  discrete delay1 : Subsystem  TreatAsAtomicUnit=on
      settings: MinAlgLoopOccurrences=on
  discrete delay2 : Subsystem  TreatAsAtomicUnit=on
      settings: MinAlgLoopOccurrences=on
  x_SS : Constant  Value=step_width-DS_width
  x_SS1 : Constant  Value=step_width-DS_width
  x_SS2 : Constant  Value=0
  Rtau_B_des [Nm] : Outport  InitialOutput=0
  Rtau_F_des [Nm] : Outport  Port=2  InitialOutput=0
  Ltau_B_des [Nm] : Outport  Port=3  InitialOutput=0
  Ltau_F_des [Nm] : Outport  Port=4  InitialOutput=0
  tag scope: Lcom_err_SS=global, Lddgamma_swing=global, Lddl_leg_swing=global, Ldgamma_swing=global, Ldl_leg_swing=global, Lgamma_swing=global, Lgrf_SS=global, Ll_leg_swing=global, Lleg_force_hip_torque_SS=global, Lshin_ctrl_trq_DS=global, Lshin_ctrl_trq_SS=global, Lshin_ctrl_trq_flight=global, Lshin_ctrl_trq_swing=global, Lthigh_ctrl_trq_DS=global, Lthigh_ctrl_trq_SS=global, Lthigh_ctrl_trq_flight=global, Lthigh_ctrl_trq_swing=global, Lvmc_kkt_cost_SS=global, Rcom_err_SS=global, Rddgamma_swing=global, Rddl_leg_swing=global, Rdgamma_swing=global, Rdl_leg_swing=global, Rgamma_swing=global, Rgrf_SS=global, Rl_leg_swing=global, Rleg_force_hip_torque_SS=global, Rshin_ctrl_trq_DS=global, Rshin_ctrl_trq_SS=global, Rshin_ctrl_trq_flight=global, Rshin_ctrl_trq_swing=global, Rthigh_ctrl_trq_DS=global, Rthigh_ctrl_trq_SS=global, Rthigh_ctrl_trq_flight=global, Rthigh_ctrl_trq_swing=global, Rvmc_kkt_cost_SS=global, com_err_DS=global, grf_DS=global, leg_force_hip_torque_DS=global, vmc_kkt_cost_DS=global
  wires:
  KKT_DS/3(grf) -> [grf_DS], discrete delay/1(t)
  [Lsplay] -> KKT_DS/10(L_splay)
  [Rsplay] -> KKT_DS/9(R_splay)
  [ddtheta_des] -> KKT_DS/3(ddtheta_des)
  [ddy_des] -> KKT_DS/2(ddy_des)
  [ddx_des] -> KKT_DS/1(ddx_des)
  discrete delay/1(t-1) -> KKT_DS/18(grf_prev)
  Demux7/1 -> Rtau_B_des [Nm]/1
  Demux7/3 -> Ltau_B_des [Nm]/1
  Demux7/4 -> Ltau_F_des [Nm]/1
  Demux7/2 -> Rtau_F_des [Nm]/1
  KKT_DS/2(leg_force_hip_torque) -> [leg_force_hip_torque_DS]
  KKT_DS/5(err) -> [com_err_DS]
  KKT_DS/4(cost_tie_break) -> [vmc_kkt_cost_DS]
  [RLength] -> KKT_DS/4(R_leg_length)
  [LLength] -> KKT_DS/5(L_leg_length)
  [theta] -> KKT_DS/11(theta)
  KKT_SS/3(grf) -> discrete delay1/1(t), [Rgrf_SS]
  [theta] -> KKT_SS/7(theta)
  Constant3/1 -> KKT_DS/12(lambda1)
  Constant4/1 -> KKT_DS/13(lambda2)
  Constant5/1 -> KKT_DS/14(lambda3)
  Constant6/1 -> KKT_SS/8(lambda1)
  Constant7/1 -> KKT_SS/9(lambda2)
  Constant8/1 -> KKT_SS/10(lambda3)
  [ddx_des] -> KKT_SS/1(ddx_des)
  [ddy_des] -> KKT_SS/2(ddy_des)
  [ddtheta_des] -> KKT_SS/3(ddtheta_des)
  KKT_DS/1(motor_trq) -> Demux8/1
  Demux8/1 -> [Rshin_ctrl_trq_DS]
  Demux8/3 -> [Lshin_ctrl_trq_DS]
  Demux8/4 -> [Lthigh_ctrl_trq_DS]
  Demux8/2 -> [Rthigh_ctrl_trq_DS]
  KKT_SS/1(motor_trq) -> Demux9/1
  Demux9/2 -> [Rthigh_ctrl_trq_SS]
  Demux9/1 -> [Rshin_ctrl_trq_SS]
  KKT_SS/2(leg_force_hip_torque) -> [Rleg_force_hip_torque_SS]
  KKT_SS/4(cost_tie_break) -> [Rvmc_kkt_cost_SS]
  KKT_SS/5(err) -> [Rcom_err_SS]
  [Rshin_ctrl_trq_swing] -> Mux19/1
  [Rthigh_ctrl_trq_swing] -> Mux19/2
  Switch1/1 -> Switch5/1
  [Rshin_ctrl_trq_SS] -> Mux21/1
  [Rthigh_ctrl_trq_SS] -> Mux21/2
  Mux19/1 -> Switch5/3
  Mux21/1 -> Switch1/1
  [Rsplay] -> KKT_SS/6(splay)
  [RLength] -> KKT_SS/4(L)
  [Rgamma] -> KKT_SS/5(gamma)
  [Ldgear_shin] -> Mux28/2
  [Lgear_shin] -> Mux28/1
  Mux28/1 -> Swing Leg Behavior3/1(Swing Back Gear [rad rad/s])
  [Rgamma] -> KKT_DS/7(R_gamma)
  [Lgamma] -> KKT_DS/8(L_gamma)
  [Ldgear_thigh] -> Mux24/2
  [Lgear_thigh] -> Mux24/1
  Mux24/1 -> Swing Leg Behavior3/2(Swing Front Gear [rad rad/s])
  [Rgamma] -> Swing Leg Behavior3/3(Stance Leg Angle [rad])
  Swing Leg Behavior3/1(Secondary Back/Front Motor Torque [Nm Nm]) -> Demux4/1
  Demux4/2 -> [Lthigh_ctrl_trq_swing]
  Demux4/1 -> [Lshin_ctrl_trq_swing]
  [Rstance_VMC] -> Logical Operator1/1
  [Rstance_VMC] -> Logical Operator/1
  [Lstance_VMC] -> Logical Operator/2
  Logical Operator/1 -> Switch3/2
  [Rthigh_ctrl_trq_DS] -> Mux7/2
  [Rshin_ctrl_trq_DS] -> Mux7/1
  Mux7/1 -> Switch3/1
  From120/1 -> Mux39/2
  From44/1 -> Mux39/1
  Mux39/1 -> Flight PD/1(R Back Gear [rad rad/s])
  From124/1 -> Mux40/2
  From123/1 -> Mux40/1
  Mux40/1 -> Flight PD/2(R Front Gear [rad rad/s])
  From126/1 -> Mux41/2
  From125/1 -> Mux41/1
  Mux41/1 -> Flight PD/3(L Back Gear [rad rad/s])
  From128/1 -> Mux42/2
  From127/1 -> Mux42/1
  Mux42/1 -> Flight PD/4(L Front Gear [rad rad/s])
  Flight PD/1(R cmd [Nm] [back front]) -> Demux14/1
  Demux14/2 -> Goto27/1
  Demux14/1 -> Goto62/1
  Flight PD/2(L cmd [Nm] [back front]) -> Demux15/1
  Demux15/2 -> Goto75/1
  Demux15/1 -> Goto76/1
  discrete delay1/1(t-1) -> KKT_SS/13(grf_prev)
  Constant14/1 -> KKT_DS/15(lambda4)
  Constant15/1 -> KKT_DS/16(mu_s)
  Constant17/1 -> KKT_SS/12(mu_s)
  Constant19/1 -> KKT_SS/11(lambda4)
  x_SS/1 -> Swing Leg Behavior3/4(Horizontal Single Support Distance [m])
  [LLength] -> Swing Leg Behavior3/5(Swing Leg Length [m])
  [dx_com] -> Swing Leg Behavior3/7(COM Forward Velocity [m/s])
  [dtheta] -> Mux31/2
  [theta] -> Mux31/1
  Mux31/1 -> Swing Leg Behavior3/8(theta [rad rad/s])
  [RtauB] -> Mux47/1
  [RtauF] -> Mux47/2
  [LtauB] -> Mux47/3
  [LtauF] -> Mux47/4
  Mux47/1 -> KKT_DS/17(sea_trqs)
  Constant23/1 -> KKT_DS/6(min_Fy)
  KKT_SS1/3(grf) -> discrete delay2/1(t), [Lgrf_SS]
  [theta] -> KKT_SS1/7(theta)
  Constant27/1 -> KKT_SS1/8(lambda1)
  Constant28/1 -> KKT_SS1/9(lambda2)
  Constant29/1 -> KKT_SS1/10(lambda3)
  [ddx_des] -> KKT_SS1/1(ddx_des)
  [ddy_des] -> KKT_SS1/2(ddy_des)
  [ddtheta_des] -> KKT_SS1/3(ddtheta_des)
  KKT_SS1/1(motor_trq) -> Demux17/1
  Demux17/2 -> [Lthigh_ctrl_trq_SS]
  Demux17/1 -> [Lshin_ctrl_trq_SS]
  KKT_SS1/2(leg_force_hip_torque) -> [Lleg_force_hip_torque_SS]
  KKT_SS1/4(cost_tie_break) -> [Lvmc_kkt_cost_SS]
  KKT_SS1/5(err) -> [Lcom_err_SS]
  [Lsplay] -> KKT_SS1/6(splay)
  [LLength] -> KKT_SS1/4(L)
  [Lgamma] -> KKT_SS1/5(gamma)
  discrete delay2/1(t-1) -> KKT_SS1/13(grf_prev)
  Constant25/1 -> KKT_SS1/12(mu_s)
  Constant26/1 -> KKT_SS1/11(lambda4)
  [Rdgear_shin] -> Mux26/2
  [Rgear_shin] -> Mux26/1
  [Rdgear_thigh] -> Mux53/2
  [Rgear_thigh] -> Mux53/1
  Mux53/1 -> Swing Leg Behavior2/2(Swing Front Gear [rad rad/s])
  Demux11/2 -> [Rthigh_ctrl_trq_swing]
  Demux11/1 -> [Rshin_ctrl_trq_swing]
  x_SS1/1 -> Swing Leg Behavior2/4(Horizontal Single Support Distance [m])
  [RLength] -> Swing Leg Behavior2/5(Swing Leg Length [m])
  [Rgamma] -> Swing Leg Behavior2/6(Swing Leg Angle [rad])
  [dx_com] -> Swing Leg Behavior2/7(COM Forward Velocity [m/s])
  [dtheta] -> Mux52/2
  [theta] -> Mux52/1
  Mux52/1 -> Swing Leg Behavior2/8(theta [rad rad/s])
  [Lgamma] -> Swing Leg Behavior3/6(Swing Leg Angle [rad])
  [Lgamma] -> Swing Leg Behavior2/3(Stance Leg Angle [rad])
  Mux26/1 -> Swing Leg Behavior2/1(Swing Back Gear [rad rad/s])
  Swing Leg Behavior3/2(Desired Leg Length [m]) -> [Ll_leg_swing]
  Swing Leg Behavior3/3(Desired Leg Length Velocity [m/s]) -> [Ldl_leg_swing]
  Swing Leg Behavior3/4(Desired Leg Length Acceleration [m/s^2]) -> [Lddl_leg_swing]
  Swing Leg Behavior3/5(Desired Global Leg Angle [m]) -> [Lgamma_swing]
  Swing Leg Behavior3/6(Desired Global Leg Angle Velocity [m/s]) -> [Ldgamma_swing]
  Swing Leg Behavior3/7(Desired Global Leg Angle Acceleration [m/s^2]) -> [Lddgamma_swing]
  [Lstance_VMC] -> Swing Leg Behavior3/9(Swing Leg Stance (VMC) [0/1])
  [Rstance_VMC] -> Swing Leg Behavior2/9(Swing Leg Stance (VMC) [0/1])
  Swing Leg Behavior2/1(Secondary Back/Front Motor Torque [Nm Nm]) -> Demux11/1
  Swing Leg Behavior2/2(Desired Leg Length [m]) -> [Rl_leg_swing]
  Swing Leg Behavior2/3(Desired Leg Length Velocity [m/s]) -> [Rdl_leg_swing]
  Swing Leg Behavior2/4(Desired Leg Length Acceleration [m/s^2]) -> [Rddl_leg_swing]
  Swing Leg Behavior2/5(Desired Global Leg Angle [m]) -> [Rgamma_swing]
  Swing Leg Behavior2/6(Desired Global Leg Angle Velocity [m/s]) -> [Rdgamma_swing]
  Swing Leg Behavior2/7(Desired Global Leg Angle Acceleration [m/s^2]) -> [Rddgamma_swing]
  Logical Operator1/1 -> Switch1/2
  From77/1 -> ?
  Switch3/1 -> Switch1/3
  Mux25/1 -> Demux7/1
  [Rshin_ctrl_trq_flight] -> Mux60/1
  [Rthigh_ctrl_trq_flight] -> Mux60/2
  Mux60/1 -> Switch3/3
  Logical Operator7/1 -> Logical Operator1/2
  [Lstance_VMC] -> Logical Operator7/1
  [Rstance_VMC] -> Switch5/2
  Switch5/1 -> Mux25/1
  [Lshin_ctrl_trq_swing] -> Mux20/1
  [Lthigh_ctrl_trq_swing] -> Mux20/2
  Switch2/1 -> Switch6/1
  [Lshin_ctrl_trq_SS] -> Mux22/1
  [Lthigh_ctrl_trq_SS] -> Mux22/2
  Mux20/1 -> Switch6/3
  Mux22/1 -> Switch2/1
  [Lstance_VMC] -> Logical Operator3/1
  [Lstance_VMC] -> Logical Operator2/1
  [Rstance_VMC] -> Logical Operator2/2
  Logical Operator2/1 -> Switch4/2
  [Lthigh_ctrl_trq_DS] -> Mux43/2
  [Lshin_ctrl_trq_DS] -> Mux43/1
  Mux43/1 -> Switch4/1
  Logical Operator3/1 -> Switch2/2
  From131/1 -> ?
  Switch4/1 -> Switch2/3
  [Lshin_ctrl_trq_flight] -> Mux23/1
  [Lthigh_ctrl_trq_flight] -> Mux23/2
  Mux23/1 -> Switch4/3
  Logical Operator4/1 -> Logical Operator3/2
  [Rstance_VMC] -> Logical Operator4/1
  [Lstance_VMC] -> Switch6/2
  Switch6/1 -> Mux25/2
  Constant24/1 -> Mux61/1
  Constant11/1 -> Mux61/2
  Constant31/1 -> Mux61/3
  Constant30/1 -> Mux61/4
  From132/1 -> Switch7/2
  Mux61/1 -> Switch7/3
  Constant39/1 -> Mux62/1
  Constant43/1 -> Mux62/2
  Constant40/1 -> Mux62/3
  Constant44/1 -> Mux62/4
  Mux62/1 -> Switch7/1
  Switch7/1 -> Demux20/1
  Demux20/1 -> Flight PD/5(R Length des [m])
  Demux20/2 -> Flight PD/6(R Gamma des [m])
  Demux20/3 -> Flight PD/7(L Length des [m])
  Demux20/4 -> Flight PD/8(L Angle des [m])
  From177/1 -> Flight PD/9(theta [rad])
  x_SS2/1 -> [Lthigh_ctrl_trq_flight], [Lshin_ctrl_trq_flight], [Rthigh_ctrl_trq_flight], [Rshin_ctrl_trq_flight]

== system ATRIAS_vnmc/control/Virtual Neuromuscular Control ==
  note: High-Level
      | Control
  note: Neural
      | Control
  note: Muscle
      | Dynamics
  note: Jacobian Mapping
  Higher Control Layer : Subsystem
  Muscle Layer : Subsystem
  Neural Control Layer1 : Subsystem
  Torque Distribution : Subsystem
  RtauB_des [Nm] : Outport
  RtauF_des [Nm] : Outport  Port=2
  LtauB_des [Nm] : Outport  Port=3
  LtauF_des [Nm] : Outport  Port=4
  tag scope: Jinv_trans_L=global, Jinv_trans_R=global
  wires:
  Torque Distribution/6(L J_inv_transpose [2x2]) -> [Jinv_trans_L]
  Torque Distribution/5(L tauF [Nm]) -> LtauF_des [Nm]/1
  Torque Distribution/4(L tauB [Nm]) -> LtauB_des [Nm]/1
  Torque Distribution/3(R J_inv_transpose [2x2]) -> [Jinv_trans_R]
  [LM12] -> Torque Distribution/4(L tauK_des [Nm])
  [LM23] -> Torque Distribution/5(L tauH_des [Nm])
  [k_R] -> Torque Distribution/3(R Jacobian Constant (k))
  [k_L] -> Torque Distribution/6(L Jacobian Constant (k))
  Torque Distribution/1(R tauB [Nm]) -> RtauB_des [Nm]/1
  Torque Distribution/2(R tauF [Nm]) -> RtauF_des [Nm]/1
  [RM23] -> Torque Distribution/2(R tauH_des [Nm])
  [RM12] -> Torque Distribution/1(R tauK_des [Nm])

== system ATRIAS_vnmc/atrias_system/ATRIAS Mechanical System Layer/Boom ==
  CS1 to CS2 : sm_lib/Frames and Transforms/Rigid Transform  TranslationMethod=Cartesian  TranslationLengthUnit=m  TranslationStandardAxis=+Z  TranslationStandardOffset=0  TranslationCartesianOffset=boom_12  TranslationROffset=0  TranslationROffsetUnits=m  TranslationZOffset=0  TranslationZOffsetUnits=m  TranslationThetaOffset=0  TranslationThetaOffsetUnits=deg  RotationMethod=None  RotationAngleUnits=deg  RotationStandardAxis=+Z  RotationAngle=0  RotationArbitraryAxis=[0 0 1]  FollAlignAxisA=+X  BaseAlignAxisA=+Y  FollAlignAxisB=+Y  BaseAlignAxisB=+Z  RotationMatrix=[1 0 0; 0 1 0; 0 0 1]  BlockFunction=simmechanics.library.frames_transforms.rigid_transform
  Frame Data : Subsystem
  Solid : sm_lib/Body Elements/Solid  InertiaType=Custom  Mass=m_boom  MassUnits=kg  CenterOfMass=com_boom  CenterOfMassUnits=m  MomentsOfInertia=i_boom_moments  MomentsOfInertiaUnits=kg*m^2  ProductsOfInertia=i_boom_products  ProductsOfInertiaUnits=kg*m^2  DensityBased=on  Density=1000  DensityUnits=kg/(m^3)  GraphicType=FromGeometry  MarkerShape=Sphere  MarkerSize=10  MarkerSizeUnits=m  GraphicVisPropType=AdvancedVisualProperties  GraphicDiffuseColor=boom_color_d  GraphicSpecularColor=[0.5 0.5 0.5 1.0]  GraphicAmbientColor=[boom_color_d*0.5 1.0]  GraphicEmissiveColor=[0.0 0.0 0.0 1.0]  GraphicShininess=128  GraphicOpacity=1.0  GeometryShape=FromFile  RectangleSize=[1 1]  RectangleSizeUnits=m  BrickDimensions=[1 1 1]  BrickDimensionUnits=m  CylinderRadius=l_rad  CylinderRadiusUnits=m  CylinderLength=l_seg  CylinderLengthUnits=m  SphereRadius=1  SphereRadiusUnits=m  EllipsoidRadii=[1 1 1]  EllipsoidRadiiUnits=m  ExtrusionCrossSection=[1 1; -1 1; -1 -1; 1 -1]  ExtrusionCrossSectionUnits=m  ExtrusionLength=1  ExtrusionLengthUnits=m  PolygonNumSides=3  PolygonOuterRadius=1  PolygonOuterRadiusUnits=m  ExtGeomFileType=STL  ExtGeomFileName=../0_images/models/boom_roll.stl  ExtGeomFileUnits=m  RevolutionCrossSection=[1 1; 1 -1; 2 -1; 2 1]  RevolutionCrossSectionUnits=m  RevolutionExtent=Full  RevolutionAngle=180  RevolutionAngleUnits=deg  BlockFunction=simmechanics.library.body_elements.solid
  CS1 : PMIOPort  Port=1  Side=Left
  CS2 : PMIOPort  Port=2  Side=Right
  connections:
  CS1/RConn1 -- Frame Data/LConn1 -- CS1 to CS2/LConn1 -- Solid/RConn1
  CS2/RConn1 -- CS1 to CS2/RConn1
